simulink model "untitled"  (R2020b)
settings: Solver=VariableStepAuto  StartTime=0.0  StopTime=100  RelTol=1e-3
settings Model: Creator=sofia  LastModifiedBy=sofia

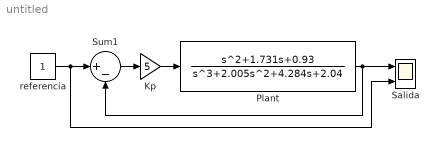
== system untitled ==
  Kp : Gain  Gain=5
  Plant : TransferFcn  Numerator=[1 1.731 0.93]  Denominator="[1  2.005 4.284 2.04]"
  Salida : Scope  NumInputPorts=2
  Sum1 : Sum  Inputs=|+-
  referencia : Constant
  wires:
  referencia/1 -> Salida/2, Sum1/1
  Plant/1 -> Salida/1, Sum1/2
  Kp/1 -> Plant/1
  Sum1/1 -> Kp/1
